simulink model "controllers"  (R2022a)
settings: Solver=FixedStepDiscrete  StartTime=0.0  StopTime=30  FixedStep=1  RelTol=1e-3  EnableMultiTasking=on
settings Model: ExtModeTrigDuration=2  Creator=Amin  LastModifiedBy=dmenr
settings SolverCC: AlgebraicLoopSolver=TrustRegion
settings OptimizationCC: DefaultParameterBehavior=Inlined  UseDivisionForNetSlopeComputation=on  GainParamInheritBuiltInType=on  UseFloatMulNetSlope=on  InlineInvariantSignals=on  PassReuseOutputArgsAs=Individual arguments  ZeroExternalMemoryAtStartup=off  ZeroInternalMemoryAtStartup=off  NoFixptDivByZeroProtection=on  EfficientFloat2IntCast=on  LifeSpan=1  MaxStackSize=64  OptimizeBlockOrder=speed  DifferentSizesBufferReuse=on  EfficientTunableParamExpr=on
settings DebuggingCC: ParameterTunabilityLossMsg=error  UnconnectedInputMsg=warning  UnconnectedOutputMsg=warning  UnconnectedLineMsg=warning  SFMachineParentedDataDiag=warning
settings HardwareCC: ProdBitPerInt=16  ProdBitPerPointer=16  ProdBitPerSizeT=16  ProdBitPerPtrDiffT=16  ProdLargestAtomicFloat=None  ProdWordSize=8  ProdLongLongMode=on  ProdHWDeviceType=Atmel->AVR
settings SFSimCC: MATLABDynamicMemAlloc=off
settings RTWCC: SystemTargetFile=ert.tlc  HardwareBoard=Arduino Mega 2560  GenCodeOnly=on  TemplateMakefile=ert_default_tmf  Toolchain=Arduino AVR  BuildConfiguration=Faster Runs
settings CodeAppCC: ForceParamTrailComments=on  IgnoreCustomStorageClasses=off  OperatorAnnotations=on  SimulinkDataObjDesc=on  SFDataObjDesc=on  CustomSymbolStrGlobalVar=rt$N$M  CustomSymbolStrType=$N$M  CustomSymbolStrFcn=$N$M$F  CustomSymbolStrMacro=$N$M  InsertBlockDesc=on
settings ERTTargetCC: IncludeMdlTerminateFcn=off  CombineSignalStateStructs=on  SupportAbsoluteTime=off  PurelyIntegerCode=on  SupportComplex=off  SupportNonInlinedSFcns=on  ExtModeStaticAllocSize=2048  InlinedParameterPlacement=NonHierarchical  ERTFilePackagingFormat=CompactWithDataFile  IndentSize=4

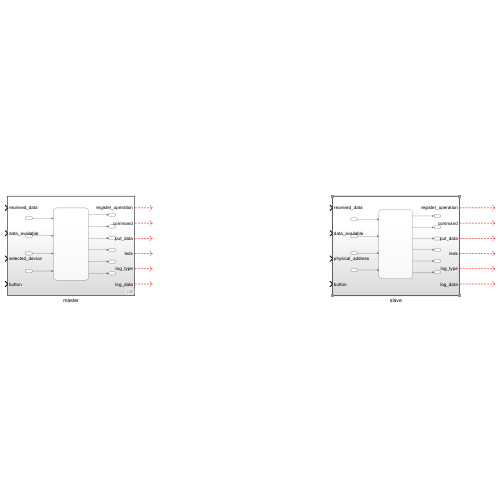
[thumbnail: Simulink's stored preview of the top-level diagram]
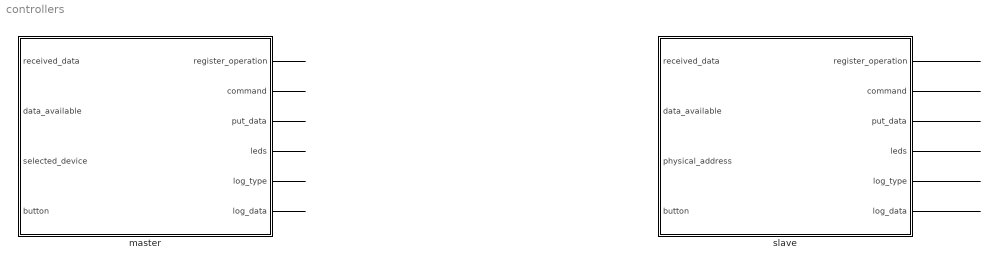
== system controllers ==
  master : Subsystem
  slave : Subsystem
  wires:
  master/1(register_operation) -> ?
  master/2(command) -> ?
  master/3(put_data) -> ?
  master/4(leds) -> ?
  slave/1(register_operation) -> ?
  slave/2(command) -> ?
  slave/3(put_data) -> ?
  slave/4(leds) -> ?
  master/5(log_type) -> ?
  master/6(log_data) -> ?
  slave/5(log_type) -> ?
  slave/6(log_data) -> ?

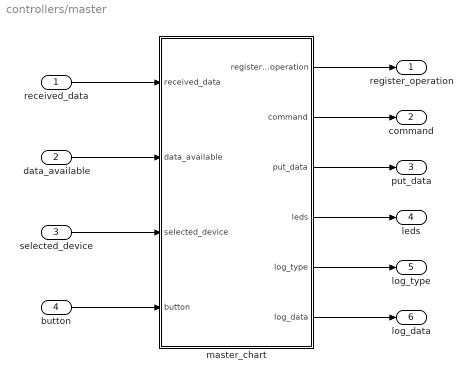
== system controllers/master ==
  received_data : Inport
  data_available : Inport  Port=2
  selected_device : Inport  Port=3
  button : Inport  Port=4
  master_chart : Stateflow chart  TreatAsAtomicUnit=on
      settings: PortSchema="{\"entries\":[{\"content\":{\"sides\":[{\"content\":{\"connectorIds\":[\"In1\",\"In2\",\"In3\",\"In4\"]},\"type\":\"ConnectorPlacement.EquallySpacedRectSide\",\"uuid\":\"138602be-6c58-4e8c-ba48-a14eddddc67c\"},{\"content\":{\"connectorIds\":[\"Out2\",\"Out1\",\"Out3\",\"Out6\",\"Out4\",\"Out5\"],\"side\":\"RIGHT\"},\"type\":\"ConnectorPlacement.EquallySpacedRectSide\",\"uuid\":\"5ecf324f-f194-43dd-983a-d068392304a8\"},{\"content\":{\"connectorIds\":[],\"side\":\"TOP\"},\"type\":\"ConnectorPlacement.EquallySpacedRectSide\",\"uuid\":\"4d10d79f-a1db-44f1-98c5-6d0be9e5b6d6\"}]},\"type\":\"ConnectorPlacement.EquallySpacedConnector\",\"uuid\":\"447fba48-e554-4a4b-a9f0-a545df5fe3d2\"}],\"packageUris\":[\"http://schema.mathworks.com/mf0/Connector/19700101\"],\"version\":\"1.0\"}"
  register_operation : Outport
  command : Outport  Port=2
  put_data : Outport  Port=3  OutDataTypeStr=uint8
  leds : Outport  Port=4
  log_type : Outport  Port=5
  log_data : Outport  Port=6
  wires:
  received_data/1 -> master_chart/1(received_data)
  master_chart/1(command) -> command/1
  data_available/1 -> master_chart/2(data_available)
  master_chart/2(register_operation) -> register_operation/1
  master_chart/3(put_data) -> put_data/1
  master_chart/4(log_type) -> log_type/1
  master_chart/5(log_data) -> log_data/1
  selected_device/1 -> master_chart/3(selected_device)
  button/1 -> master_chart/4(button)
  master_chart/6(leds) -> leds/1

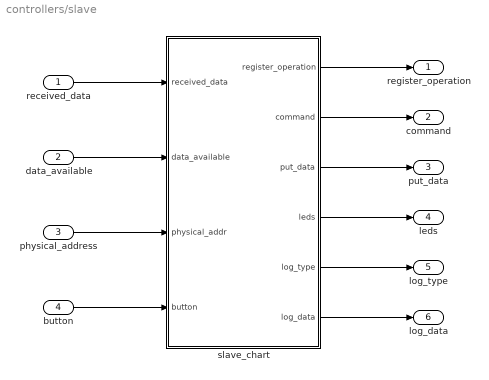
== system controllers/slave ==
  received_data : Inport
  data_available : Inport  Port=2
  physical_address : Inport  Port=3
  button : Inport  Port=4
  slave_chart : Stateflow chart  TreatAsAtomicUnit=on
      settings: PortSchema="{\"entries\":[{\"content\":{\"sides\":[{\"content\":{\"connectorIds\":[\"In1\",\"In2\",\"In3\",\"In4\"]},\"type\":\"ConnectorPlacement.EquallySpacedRectSide\",\"uuid\":\"138602be-6c58-4e8c-ba48-a14eddddc67c\"},{\"content\":{\"connectorIds\":[\"Out2\",\"Out1\",\"Out3\",\"Out6\",\"Out4\",\"Out5\"],\"side\":\"RIGHT\"},\"type\":\"ConnectorPlacement.EquallySpacedRectSide\",\"uuid\":\"5ecf324f-f194-43dd-983a-d068392304a8\"},{\"content\":{\"connectorIds\":[],\"side\":\"TOP\"},\"type\":\"ConnectorPlacement.EquallySpacedRectSide\",\"uuid\":\"4d10d79f-a1db-44f1-98c5-6d0be9e5b6d6\"}]},\"type\":\"ConnectorPlacement.EquallySpacedConnector\",\"uuid\":\"447fba48-e554-4a4b-a9f0-a545df5fe3d2\"}],\"packageUris\":[\"http://schema.mathworks.com/mf0/Connector/19700101\"],\"version\":\"1.0\"}"
  register_operation : Outport
  command : Outport  Port=2
  put_data : Outport  Port=3  OutDataTypeStr=uint8
  leds : Outport  Port=4  OutDataTypeStr=uint8
  log_type : Outport  Port=5
  log_data : Outport  Port=6
  wires:
  received_data/1 -> slave_chart/1(received_data)
  slave_chart/1(command) -> command/1
  data_available/1 -> slave_chart/2(data_available)
  slave_chart/2(register_operation) -> register_operation/1
  slave_chart/3(put_data) -> put_data/1
  physical_address/1 -> slave_chart/3(physical_addr)
  slave_chart/4(log_type) -> log_type/1
  slave_chart/5(log_data) -> log_data/1
  slave_chart/6(leds) -> leds/1
  button/1 -> slave_chart/4(button)

== stateflow chart controllers/slave/slave_chart ==
  settings: updateMethod=DISCRETE  sampleTime=1
  state startup
    entry:
    command = SlaveCommand.SLAVE_IDLE;
    log_type = Log.LOG_NOTHING;
    leds = 0;
    button_old = 0;
  state update_leds
    entry:
    command = SlaveCommand.SLAVE_IDLE;
    log_type = Log.LOG_BUTTON_PRESSED;
    log_data[0] = button_pressed(button_old, button);
    leds = leds ^ (button ^ button_old);
    button_old = button;
    during:
    exit:
    log_type = Log.LOG_NOTHING;
  state result  = button_pressed(old_state, current_state) [function]
    (default) -> (junction 336)
    (junction 336) -> (junction 334) : {result = 0}
    (junction 334) -> (junction 333) [order 1] : [result < sizeof(old_state)]
    (junction 333) -> (junction 334) [order 2] : {result = result + 1}
    (junction 333) -> (junction 331) [order 1] : [old_state[result] == 0 && current_state[result] == 1]
    (junction 334) -> (junction 331) [order 2]
  state bus_idle
    entry:
    register_operation = Operation.OPERATION_READ;
    command = SlaveCommand.SLAVE_READ;
    log_type = Log.LOG_NOTHING;
    during:
    button_old = button
    exit:
  state read_register_address
    entry:
    register_operation = Operation.OPERATION_READ;
    command = SlaveCommand.SLAVE_READ;
    during:
    exit:
  state wait_bus_idle
    entry:
    register_operation = Operation.OPERATION_READ;
    command = SlaveCommand.SLAVE_IGNORE;
    button_old = button
    idle_clocks = 0;
    during:
    idle_clocks = idle_clocks + 1;
    exit:
  state results  = extract_bits(data) [function]
    (default) -> (junction 363)
    (junction 363) -> (junction 365) : {i = 0;}
    (junction 365) -> (junction 368) [order 1] : [i < sizeof(results)]
    (junction 366) -> (junction 365) : {i = i + 1;}
    (junction 368) -> (junction 366) : {results[i] = data & 0x1;
        | data = data >> 1;}
    (junction 365) -> (junction 364) [order 2]
  state wait_for_master
    entry:
    command = SlaveCommand.SLAVE_IDLE;
    during:
    exit:
  state read_data
    entry:
    register_operation = Operation.OPERATION_READ;
    command = SlaveCommand.SLAVE_READ;
    during:
    exit:
  state put_data
    entry:
    register_operation = Operation.OPERATION_WRITE;
    command = SlaveCommand.SLAVE_PUT;
    put_data = combine_bits(leds)
    log_type = Log.LOG_REPLY;
    log_data[0] = put_data;
    during:
    exit:
  state output  = combine_bits(bits) [function]
    (default) -> (junction 351)
    (junction 351) -> (junction 352) : {i = 0; output = 0}
    (junction 352) -> (junction 356) [order 1] : [i < sizeof(bits)]
    (junction 344) -> (junction 352) : {i = i + 1;}
    (junction 356) -> (junction 344) : {output |= bits[i] << i;}
    (junction 352) -> (junction 346) [order 2]
  state process_data
    entry:
    command = SlaveCommand.SLAVE_IDLE;
    log_type = Log.LOG_RECEIVE;
    log_data[0] = 0;
    log_data[1] = received_data;
    leds =extract_bits(received_data);
    during:
    exit:
  (default) -> startup
  update_leds -> update_leds [order 1] : [button_pressed(button_old, button) != sizeof(button)]
  startup -> bus_idle : [true]
  bus_idle -> update_leds [order 3] : [button_pressed(button_old, button) != sizeof(button)]{from_wait_bus = false}
  bus_idle -> read_register_address [order 1] : [data_available == true && received_data == physical_addr]
  update_leds -> bus_idle [order 2] : [from_wait_bus == false]
  (junction 107) -> bus_idle
  wait_bus_idle -> bus_idle [order 1] : [idle_clocks >= 3]
  bus_idle -> wait_bus_idle [order 2] : [data_available == true && received_data != physical_addr]
  update_leds -> wait_bus_idle [order 3] : [from_wait_bus == true]
  wait_bus_idle -> update_leds [order 2] : [button_pressed(button_old, button) != sizeof(button)]{from_wait_bus = true}
  read_register_address -> wait_for_master : [data_available == true]
  wait_bus_idle -> wait_bus_idle [order 3] : [data_available == true]{idle_clocks = 0}
  wait_for_master -> read_data [order 1] : [received_data == 0]
  wait_for_master -> put_data [order 2] : [received_data == (1 << 7) | 0]
  read_data -> process_data : [data_available == true]
  put_data -> (junction 107) : [true]
  process_data -> (junction 107) : [true]
  data: old_state function_input uint8 size=[1 8]; current_state function_input uint8 size=[1 8]; result function_output uint8; data function_input uint8; results function_output uint8 size=[1 8]; i temporary uint8; bits function_input uint8 size=[1 8]; output function_output uint8; i temporary uint8; received_data input uint8; command output Enum: SlaveCommand; data_available input boolean; register_operation output Enum: Operation; put_data output uint8; idle_clocks local uint8; physical_addr input uint8; log_type output Enum: Log; log_data output uint8 size=[1 3]; button_old local uint8 size=[1 8]; leds output uint8 size=[1 8]; button input uint8 size=[1 8]; from_wait_bus local boolean

== stateflow chart controllers/master/master_chart ==
  settings: updateMethod=DISCRETE  sampleTime=1
  state bus_idle
    entry:
    command = MasterCommand.MASTER_IDLE;
    log_type = Log.LOG_NOTHING;
    button_old = button;
    last_selected_device = selected_device;
    during:
    exit:
  state result  = button_pressed(old_state, current_state) [function]
    (default) -> (junction 180)
    (junction 180) -> (junction 173) : {result = 0}
    (junction 173) -> (junction 177) [order 1] : [result < sizeof(old_state)]
    (junction 177) -> (junction 173) [order 2] : {result = result + 1}
    (junction 177) -> (junction 175) [order 1] : [old_state[result] == 0 && current_state[result] == 1]
    (junction 173) -> (junction 175) [order 2]
  state update_leds
    entry:
    command = MasterCommand.MASTER_IDLE;
    log_type = Log.LOG_BUTTON_PRESSED;
    log_data[0] = button_pressed(button_old, button);
    leds = leds ^ (button ^ button_old);
    button_old = button;
    phy_addr = uint8(selected_device);
    reg_addr = 0;
    during:
    exit:
    log_type = Log.LOG_NOTHING;
  state retrieve_leds
    entry:
    command = MasterCommand.MASTER_IDLE;
    phy_addr = uint8(selected_device);
    reg_addr = (1 << 7) | 0;
    log_type = Log.LOG_RETRIEVE_STATE;
    log_data[0] = phy_addr;
    during:
    exit:
    log_type = Log.LOG_NOTHING;
  state results  = extract_bits(data) [function]
    (default) -> (junction 258)
    (junction 258) -> (junction 253) : {i = 0;}
    (junction 253) -> (junction 261) [order 1] : [i < sizeof(results)]
    (junction 259) -> (junction 253) : {i = i + 1;}
    (junction 261) -> (junction 259) : {results[i] = data & 0x1;
        | data = data >> 1;}
    (junction 253) -> (junction 260) [order 2]
  state send_physical_address
    entry:
    register_operation = Operation.OPERATION_WRITE;
    command = MasterCommand.MASTER_PUT;
    put_data = uint8(phy_addr);
    during:
    exit:
  state startup
    entry:
    command = MasterCommand.MASTER_IDLE;
    log_type = Log.LOG_NOTHING;
    phy_addr = uint8(selected_device);
    reg_addr = (1 << 7) | 0;
    leds = 0;
    button_old = 0;
  state output  = combine_bits(bits) [function]
    (default) -> (junction 267)
    (junction 267) -> (junction 269) : {i = 0; output = 0}
    (junction 269) -> (junction 272) [order 1] : [i < sizeof(bits)]
    (junction 270) -> (junction 269) : {i = i + 1;}
    (junction 272) -> (junction 270) : {output |= bits[i] << i;}
    (junction 269) -> (junction 268) [order 2]
  state send_register_address
    entry:
    register_operation = Operation.OPERATION_WRITE;
    command = MasterCommand.MASTER_PUT;
    put_data = reg_addr;
    during:
    exit:
  state read_data
    entry:
    register_operation = Operation.OPERATION_READ;
    command = MasterCommand.MASTER_READ;
    during:
    exit:
  state put_data
    entry:
    register_operation = Operation.OPERATION_WRITE;
    command = MasterCommand.MASTER_PUT;
    put_data = combine_bits(leds);
    log_type = Log.LOG_SEND;
    log_data[0] = phy_addr;
    log_data[1] = reg_addr;
    log_data[2] = put_data;
    during:
    exit:
  state process_data
    entry:
    command = MasterCommand.MASTER_IDLE;
    log_type = Log.LOG_RECEIVE;
    log_data[0] = phy_addr;
    log_data[1] = reg_addr;
    log_data[2] = received_data;
    leds = extract_bits(received_data)
    during:
    exit:
  state wait_bus_idle
    entry:
    command = MasterCommand.MASTER_IDLE;
    log_type = Log.LOG_NOTHING;
    idle_clocks = 0;
    during:
    idle_clocks = idle_clocks + 1;
    exit:
    retrieve_timeout = 50;
  bus_idle -> retrieve_leds [order 1] : [retrieve_timeout == 0 | last_selected_device != selected_device]
  bus_idle -> update_leds [order 2] : [button_pressed(button_old, button) != sizeof(button)]
  wait_bus_idle -> bus_idle : [idle_clocks >= 5]
  bus_idle -> bus_idle [order 3] : [retrieve_timeout > 0]{retrieve_timeout--}
  update_leds -> send_physical_address : [true]
  retrieve_leds -> send_physical_address : [true]
  (default) -> startup
  startup -> send_physical_address : [true]
  send_physical_address -> send_register_address : [true]
  send_register_address -> put_data [order 1] : [reg_addr == 0]
  send_register_address -> read_data [order 2] : [reg_addr == (1 << 7) | 0]
  read_data -> process_data : [data_available == true]
  put_data -> wait_bus_idle : [true]
  process_data -> wait_bus_idle : [true]
  data: old_state function_input uint8 size=[1 8]; current_state function_input uint8 size=[1 8]; result function_output uint8; data function_input uint8; results function_output uint8 size=[1 8]; i temporary uint8; bits function_input uint8 size=[1 8]; output function_output uint8; i temporary uint8; received_data input uint8; command output Enum: MasterCommand; data_available input boolean; register_operation output Enum: Operation; put_data output uint8; idle_clocks local uint8; phy_addr local uint8; reg_addr local uint8; log_type output Enum: Log; log_data output uint8 size=[1 3]; selected_device input uint8; leds output uint8 size=[1 8]; retrieve_timeout local uint8; button input uint8 size=[1 8]; button_old local uint8 size=[1 8]; last_selected_device local uint8
